simulink model "Simulink_detumbling_con_sensori"  (R2026a)
settings: Solver=ode5  StopTime=30000  FixedStep=0.1
values from neighbouring files (symbols this model uses):
  init_state = [init_quat'; init_angvel_rad']    [InitFeedback.m]
  k_bdot = (2 * omega_0 * (1 + sin(inc_m)) * I_min) / (B_mean^2)    [InitFeedback.m]
  Sat_Inertia = diag([7600, 8700, 5100])    [InitFeedback.m]
  Ts_gyro = 1/sample_f    (= 0.1)    [InitFeedback.m]
libraries: simulink x2
settings Model: Creator=mtt17  LastModifiedBy=mtt17

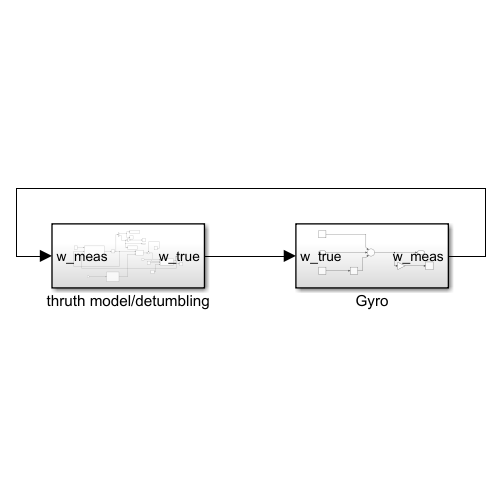
[thumbnail: Simulink's stored preview of the top-level diagram]
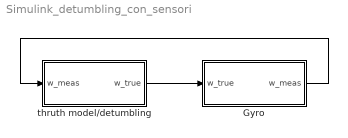
== system Simulink_detumbling_con_sensori ==
  Gyro : Subsystem
  thruth model/detumbling : Subsystem
  wires:
  thruth model/detumbling/1(w_true) -> Gyro/1(w_true)
  Gyro/1(w_meas) -> thruth model/detumbling/1(w_meas)

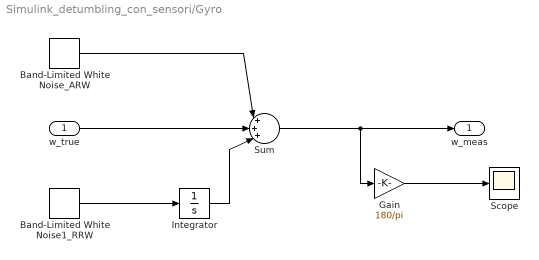
== system Simulink_detumbling_con_sensori/Gyro ==
  w_true : Inport
  Band-Limited White Noise1_RRW : simulink/Sources/Band-Limited White Noise  Cov=noise_power_RRW  Ts=Ts_gyro  seed=[4;5;6]
  Band-Limited White Noise_ARW : simulink/Sources/Band-Limited White Noise  Cov=noise_power_ARW  Ts=Ts_gyro  seed=[1; 2; 3]
  Gain : Gain  Gain=180/pi
  Integrator : Integrator  InitialCondition=[0;0;0]
  Scope : Scope
      settings: ActiveDisplayYMinimum=-5.8672822233837509  ActiveDisplayYMaximum=6.1866968817450658
  Sum : Sum  Inputs=|+++|
  w_meas : Outport
  wires:
  Band-Limited White Noise1_RRW/1 -> Integrator/1
  Integrator/1 -> Sum/3
  w_true/1 -> Sum/2
  Band-Limited White Noise_ARW/1 -> Sum/1
  Sum/1 -> Gain/1, w_meas/1
  Gain/1 -> Scope/1

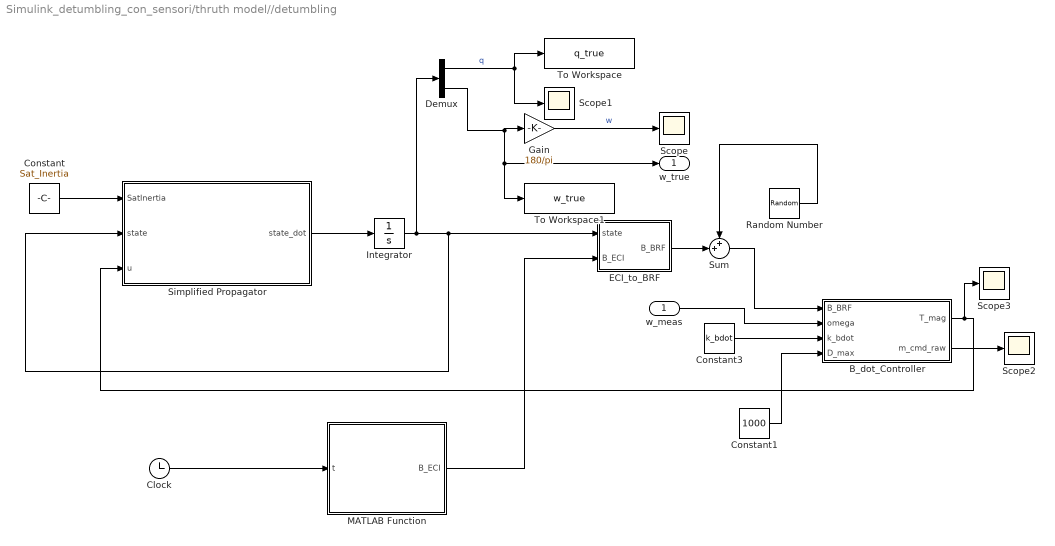
== system Simulink_detumbling_con_sensori/thruth model//detumbling ==
  w_meas : Inport
  " ECI_to_BRF" : MATLAB Function  TreatAsAtomicUnit=on
  B_dot_Controller : MATLAB Function  TreatAsAtomicUnit=on
  Clock : Clock
  Constant : Constant  Value=Sat_Inertia
  Constant1 : Constant  Value=1000
  Constant3 : Constant  Value=k_bdot
  Demux : Demux  Outputs=[4,3]
  Gain : Gain  Gain=180/pi
  Integrator : Integrator  InitialCondition=init_state
  MATLAB Function : MATLAB Function  TreatAsAtomicUnit=on
  Random Number : RandomNumber  Variance=(50e-9)^2  Seed=[1; 2; 3]  SampleTime=0.1
  Scope{,1..3} (4 alike) : Scope
      Scope settings: ActiveDisplayYMinimum=-0.13809187049764737  ActiveDisplayYMaximum=0.055531413755301462  DataLoggingVariableName=ScopeData3
      Scope1 settings: ActiveDisplayYMinimum=-0.89548652861856126  ActiveDisplayYMaximum=1.1206553324897754  DataLoggingVariableName=ScopeData4
      Scope2 settings: ActiveDisplayYMinimum=-287.67568345433358  ActiveDisplayYMaximum=30.299912549897329  DataLoggingVariableName=ScopeData5
      Scope3 settings: ActiveDisplayYMinimum=-0.0767597310270972  ActiveDisplayYMaximum=0.076218063394715888
  Simplified Propagator : MATLAB Function  TreatAsAtomicUnit=on
  Sum : Sum  Inputs=++|
  To Workspace : ToWorkspace  VariableName=q_true  SampleTime=-1
      settings: Save2DSignal=2-D array (concatenate along first dimension)
  To Workspace1 : ToWorkspace  VariableName=w_true  SampleTime=-1
      settings: Save2DSignal=2-D array (concatenate along first dimension)
  w_true : Outport
  wires:
  Simplified Propagator/1(state_dot) -> Integrator/1
  MATLAB Function/1(B_ECI) -> " ECI_to_BRF"/2(B_ECI)
  " ECI_to_BRF"/1(B_BRF) -> Sum/2
  Demux/2 -> To Workspace1/1, w_true/1, Gain/1
  Integrator/1 -> " ECI_to_BRF"/1(state), Simplified Propagator/2(state), Demux/1
  B_dot_Controller/2(m_cmd_raw) -> Scope2/1
  Constant1/1 -> B_dot_Controller/4(D_max)
  Constant/1 -> Simplified Propagator/1(SatInertia)
  Sum/1 -> B_dot_Controller/1(B_BRF)
  Clock/1 -> MATLAB Function/1(t)
  Constant3/1 -> B_dot_Controller/3(k_bdot)
  Random Number/1 -> Sum/1
  Gain/1 -> Scope/1  "w"
  Demux/1 -> Scope1/1, To Workspace/1  "q"
  w_meas/1 -> B_dot_Controller/2(omega)
  B_dot_Controller/1(T_mag) -> Scope3/1, Simplified Propagator/3(u)

== matlab function Simulink_detumbling_con_sensori/thruth model//detumbling/ ECI_to_BRF ==
  data: state input; B_BRF output; B_ECI input
function B_BRF = fcn(state, B_ECI)
    % Estrazione dei quaternioni (Convenzione Scalar-Last)
    q = state(1:4);
    q1 = q(1); q2 = q(2); q3 = q(3); q4 = q(4); % q4 è lo scalare
    
    % Matrice di rotazione da Inerziale a Body Frame (R_ECI2BRF)
    R = [q4^2+q1^2-q2^2-q3^2,   2*(q1*q2+q4*q3),     2*(q1*q3-q4*q2);
         2*(q1*q2-q4*q3),       q4^2-q1^2+q2^2-q3^2, 2*(q2*q3+q4*q1);
         2*(q1*q3+q4*q2),       2*(q2*q3-q4*q1),     q4^2-q1^2-q2^2+q3^2];
         
    % Calcolo del campo magnetico nel Body Frame
    B_BRF = R * B_ECI;
end

== matlab function Simulink_detumbling_con_sensori/thruth model//detumbling/B_dot_Controller ==
  data: B_BRF input; T_mag output; omega input; k_bdot input; D_max input; m_cmd_raw output
function [T_mag,m_cmd_raw]= fcn(B_BRF, omega, k_bdot, D_max)
    % 0. Messa in sicurezza delle dimensioni (forziamo a vettori colonna 3x1)
    B_BRF_col = [B_BRF(1); B_BRF(2); B_BRF(3)];
    omega_col = [omega(1); omega(2); omega(3)];
    
    % 1. Calcolo analitico della derivata del campo magnetico
    B_dot_BRF = -cross(omega_col, B_BRF_col);
    
    % 2. Calcolo del dipolo comandato (Usa il k_bdot dello script!)
    m_cmd_raw = -k_bdot * B_dot_BRF;

    %% 3satruazione dipendente
    m_cmd = min(max(m_cmd_raw, -D_max), D_max);
    
    %% 3. Saturazione vettoriale (Preserva la direzione del dipolo)
    % norm_m = norm(m_cmd_raw);
    % if norm_m > D_max
    %     m_cmd = m_cmd_raw * (D_max / norm_m);
    % else
    %     m_cmd = m_cmd_raw;
    % end
    % 
    %% 4. Calcolo della coppia magnetica generata
    T_mag = cross(m_cmd, B_BRF_col);
end

== matlab function Simulink_detumbling_con_sensori/thruth model//detumbling/MATLAB Function ==
  data: t input; B_ECI output
function B_ECI = fcn(t)
    % 1. Pre-allochiamo subito l'uscita in modo che Simulink conosca la dimensione!
    B_ECI = zeros(3,1);
    
    % Dichiarazione funzione esterna IGRF
    coder.extrinsic('igrfmagm');

    % 2. Pre-allochiamo anche la variabile di appoggio per l'IGRF
    B_NED_nT = zeros(3,1); 

  % Parametri Orbitali
alt  = 600;
R_E  = 6378.1363;
a    = R_E + alt;
mu   = 398600;

% Velocità angolari — PRIMA di usarle
omega_orb   = sqrt(mu / a^3);
omega_earth = (2*pi) / (24*3600);

% Elementi orbitali
inc  = 15.3 * (pi/180);
RAAN = 27.3 * (pi/180);
om   = 20.2 * (pi/180);

% Argomento di latitudine
theta = omega_orb * t + om;

% Posizione ECI con RAAN, inc, om
x_eci = a * (cos(RAAN)*cos(theta) - sin(RAAN)*sin(theta)*cos(inc));
y_eci = a * (sin(RAAN)*cos(theta) + cos(RAAN)*sin(theta)*cos(inc));
z_eci = a * sin(inc)*sin(theta);

% Latitudine e Longitudine
lat_rad = asin(z_eci / a);
lon_rad = atan2(y_eci, x_eci) - omega_earth * t;
lat = lat_rad * (180/pi);
lon = lon_rad * (180/pi);
year = 2026.4;

% IGRF
B_NED_nT = igrfmagm(alt, lat, lon, year);
    
    % Matrice di Rotazione NED -> ECEF
    sL = sin(lat_rad); cL = cos(lat_rad);
    sl = sin(lon_rad); cl = cos(lon_rad);
    
    R_NED_to_ECEF = [ -sL*cl, -sl, -cL*cl;
                      -sL*sl,  cl, -cL*sl;
                       cL,      0, -sL ];  
                       
    % Matrice di Rotazione ECEF -> ECI
    theta_g = omega_earth * t;
    st = sin(theta_g); ct = cos(theta_g);
    
    R_ECEF_to_ECI = [ ct, -st, 0;
                      st,  ct, 0;
                       0,   0, 1 ];
                       
    % Calcolo del campo in Inerziale (ECI)
    B_ECI_nT = R_ECEF_to_ECI * R_NED_to_ECEF * B_NED_nT;
    
    % Conversione in Tesla [T] per il Truth Model
    B_ECI = B_ECI_nT * 1e-9;
end

== matlab function Simulink_detumbling_con_sensori/thruth model//detumbling/Simplified Propagator ==
  data: SatInertia input; state input; u input; state_dot output
function state_dot = fcn(SatInertia, state, u)
    % Estrazione dello stato attuale
    q = state(1:4); % Quaternioni [q1; q2; q3; q4]
    w = state(5:7); % Velocità angolare [wx; wy; wz]
    
    % Matrice antisimmetrica della velocità angolare per i prodotti vettoriali
    skew_w = [  0   -w(3)  w(2);
               w(3)   0   -w(1);
              -w(2)  w(1)   0  ];
              
    % 1. DINAMICA: Equazione di Eulero per il corpo rigido
    % Calcolo della derivata della velocità angolare (w_dot)
    % Nota: 'u' è la coppia di controllo in ingresso
    w_dot = inv(SatInertia) * (u - skew_w * (SatInertia * w));
    
    % 2. CINEMATICA: Derivata dei quaternioni (Convenzione Scalar-Last)
    q_v = q(1:3); % Parte vettoriale
    q_s = q(4);   % Parte scalare
    
    q_v_dot = -0.5 * skew_w * q_v + 0.5 * q_s * w;
    q_s_dot = -0.5 * w' * q_v;
    q_dot = [q_v_dot; q_s_dot];
    
    % Vettore di stato derivato in uscita [7x1]
    state_dot = [q_dot; w_dot];
end
